simulink model "Verification_Sensors_Primitive"  (R2012b)
settings: Solver=FixedStepDiscrete  StartTime=0.0  StopTime=10.0  FixedStep=0.1  RelTol=1e-3
libraries: sldvlib x7
settings Model: Creator=Kerianne  LastModifiedBy=Kerianne
settings DataIOCC: SaveFormat=Structure
settings OptimizationCC: InlineParams=on

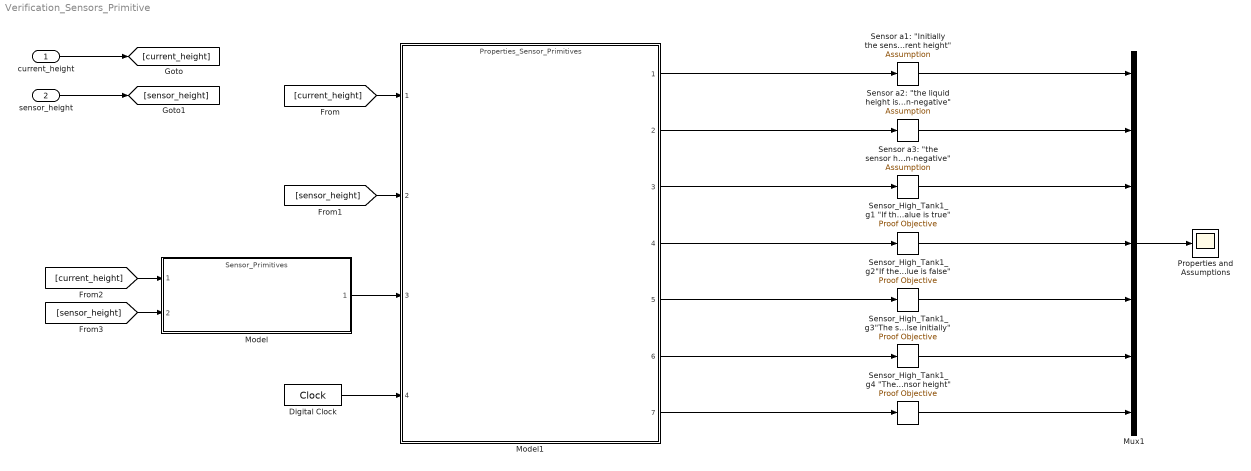
== system Verification_Sensors_Primitive ==
  current_height : Inport  OutDataTypeStr=double
  sensor_height : Inport  Port=2  OutDataTypeStr=double
  Digital Clock : DigitalClock  SampleTime=0.1
  Model : ModelReference  ModelNameDialog=Sensor_Primitives  SimulationMode=Normal  ModelReferenceVersion=1.33  CopyOfModelName=Sensor_Primitives  DefaultDataLogging=on
  Model1 : ModelReference  ModelNameDialog=Properties_Sensor_Primitives  SimulationMode=Normal  ModelReferenceVersion=1.15  CopyOfModelName=Properties_Sensor_Primitives  DefaultDataLogging=on
  Mux1 : Mux  Inputs=7
  Properties and Assumptions : Scope
      settings: ShowLegends=on
  "Sensor a1: \"Initially the sensor height is greater than the current height\"" : sldvlib/Objectives and Constraints/Assumption  enabled=on  customAVTBlockType=Assumption  intervals=true  initial=off  dispValues=on  outEnabled=on
      settings: AttributesFormatString=%<intervals>
  "Sensor a2: \"the liquid height is non-negative\"" : sldvlib/Objectives and Constraints/Assumption  enabled=on  customAVTBlockType=Assumption  intervals=true  initial=off  dispValues=on  outEnabled=on
      settings: AttributesFormatString=%<intervals>
  "Sensor a3: \"the sensor height is non-negative\"" : sldvlib/Objectives and Constraints/Assumption  enabled=on  customAVTBlockType=Assumption  intervals=true  initial=off  dispValues=on  outEnabled=on
      settings: AttributesFormatString=%<intervals>
  "Sensor_High_Tank1_g1 \"If the tank height is greater than or equal to the sensor height then Sensor_Value is true\"" : sldvlib/Objectives and Constraints/Proof Objective  enabled=on  customAVTBlockType=Proof Objective  intervals=true  dispValues=on  outEnabled=on  enableStopSim=off
      settings: AttributesFormatString=%<intervals>
  "Sensor_High_Tank1_g2\"If the tank height is less than the sensor height then Sensor_Value is false\" " : sldvlib/Objectives and Constraints/Proof Objective  enabled=on  customAVTBlockType=Proof Objective  intervals=true  dispValues=on  outEnabled=on  enableStopSim=off
      settings: AttributesFormatString=%<intervals>
  "Sensor_High_Tank1_g3\"The sensor should be false initially\"" : sldvlib/Objectives and Constraints/Proof Objective  enabled=on  customAVTBlockType=Proof Objective  intervals=true  dispValues=on  outEnabled=on  enableStopSim=off
      settings: AttributesFormatString=%<intervals>
  "Sensor_High_Tank1_g4 \"The sensor_height is the same as the specified sensor height\"" : sldvlib/Objectives and Constraints/Proof Objective  enabled=on  customAVTBlockType=Proof Objective  intervals=true  dispValues=on  outEnabled=on  enableStopSim=off
      settings: AttributesFormatString=%<intervals>
  wires:
  Mux1/1 -> Properties and Assumptions/1
  [sensor_height] -> Model1/2
  [current_height] -> Model1/1
  current_height/1 -> [current_height]
  sensor_height/1 -> [sensor_height]
  [sensor_height] -> Model/2
  [current_height] -> Model/1
  Digital Clock/1 -> Model1/4
  Model/1 -> Model1/3
  "Sensor a1: \"Initially the sensor height is greater than the current height\""/1 -> Mux1/1
  "Sensor_High_Tank1_g4 \"The sensor_height is the same as the specified sensor height\""/1 -> Mux1/7
  "Sensor_High_Tank1_g3\"The sensor should be false initially\""/1 -> Mux1/6
  "Sensor a2: \"the liquid height is non-negative\""/1 -> Mux1/2
  "Sensor a3: \"the sensor height is non-negative\""/1 -> Mux1/3
  "Sensor_High_Tank1_g1 \"If the tank height is greater than or equal to the sensor height then Sensor_Value is true\""/1 -> Mux1/4
  "Sensor_High_Tank1_g2\"If the tank height is less than the sensor height then Sensor_Value is false\" "/1 -> Mux1/5
  Model1/7 -> "Sensor_High_Tank1_g4 \"The sensor_height is the same as the specified sensor height\""/1
  Model1/6 -> "Sensor_High_Tank1_g3\"The sensor should be false initially\""/1
  Model1/5 -> "Sensor_High_Tank1_g2\"If the tank height is less than the sensor height then Sensor_Value is false\" "/1
  Model1/1 -> "Sensor a1: \"Initially the sensor height is greater than the current height\""/1
  Model1/2 -> "Sensor a2: \"the liquid height is non-negative\""/1
  Model1/3 -> "Sensor a3: \"the sensor height is non-negative\""/1
  Model1/4 -> "Sensor_High_Tank1_g1 \"If the tank height is greater than or equal to the sensor height then Sensor_Value is true\""/1
